simulink model "Control_System"  (R2018a)
settings: Solver=VariableStepAuto  StartTime=0.0  StopTime=100  RelTol=1e-3
settings Model: Creator=110116070  LastModifiedBy=110116070

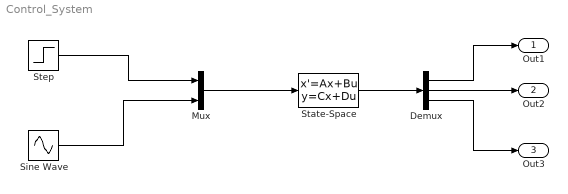
== system Control_System ==
  Demux : Demux  Outputs=3
  Mux : Mux  Inputs=2
  Sine Wave : Sin  SampleTime=0
  State-Space : StateSpace  A=[-1 -1 0; 1 -1 -1; 0 1 -1]  B=[1 0; 0 0; 0 1]  C=[-1 0 0; 0 1 0; 0 0 1]  D=[1 0; 0 0; 0 -1]  InitialCondition=0
  Step : Step  SampleTime=0
  Out1 : Outport
  Out2 : Outport  Port=2
  Out3 : Outport  Port=3
  wires:
  Step/1 -> Mux/1
  Sine Wave/1 -> Mux/2
  Mux/1 -> State-Space/1
  State-Space/1 -> Demux/1
  Demux/1 -> Out1/1
  Demux/2 -> Out2/1
  Demux/3 -> Out3/1
